simulink model "EPSAC_SM_BUCK"  (R2016a)
settings: Solver=VariableStepAuto  StartTime=0.0  StopTime=5  FixedStep=1e-5  RelTol=1e-3
libraries: powerlib x10
settings Model: Creator=jorda  LastModifiedBy=jorda

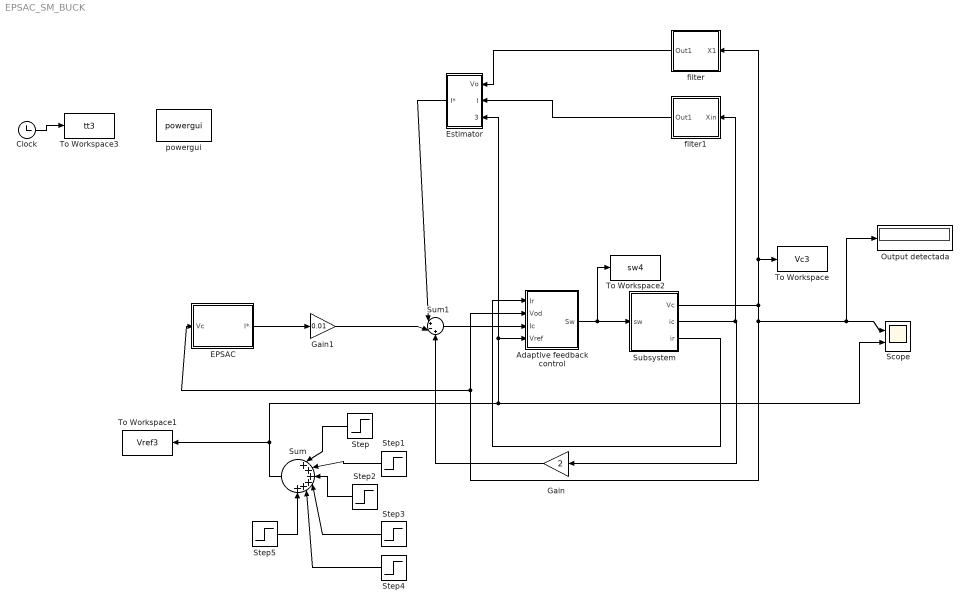
== system EPSAC_SM_BUCK ==
  "Adaptive feedback control " : Subsystem
  Clock : Clock
  EPSAC : Subsystem
  Estimator : Subsystem
  Gain : Gain  Gain=2
  Gain1 : Gain  Gain=0.01
  Output detectada : Display
  Scope : Scope  NumInputPorts=2
  Step : Step  Time=0.5  Before=3  After=4  SampleTime=0
  Step1 : Step  SampleTime=0
  Step2 : Step  Time=1.5  After=-2  SampleTime=0
  Step3 : Step  Time=2  After=-1  SampleTime=0
  Step4 : Step  Time=2.5  After=-1  SampleTime=0
  Step5 : Step  Time=3  After=2  SampleTime=0
  Subsystem : Subsystem
  Sum : Sum  Inputs=|++++++
  Sum1 : Sum  Inputs=|+-+
  To Workspace : ToWorkspace  VariableName=Vc3  SampleTime=1e-3
  To Workspace1 : ToWorkspace  VariableName=Vref3  SampleTime=1e-3
  To Workspace2 : ToWorkspace  VariableName=sw4  SampleTime=1e-3
  To Workspace3 : ToWorkspace  VariableName=tt3  SampleTime=1e-3
  filter : Subsystem
  filter1 : Subsystem
  powergui : powerlib/powergui  Priority=1  SimulationMode=Continuous  SolverType=Tustin/Backward Euler (TBE)  SampleTime=50e-6  frequency=60  SPID=off  DisableSnubberDevices=off  DisableRonSwitches=off  DisableVfSwitches=off  SwTol=0  DisplayEquations=off  Interpol=off  ExternalGateDelay=off  methode=off  Ts=10  FunctionMessages=off  echomessages=off  HookPort=off  EnableUseOfTLC=off  x0status=blocks  frequencyindice=0  Pbase=100e6  ErrMax=1e-4  Iterations=50  UnitsV=kV  UnitsW=MW  buscounter=0  RestoreLinks=warning  ResistiveCurrentMeasurement=off  Frange=[0:2:500]  Ylog=off  Xlog=on  ShowGrid=off  save=off  variable=ZData  structure=0  ZoomFFT=off  StartTime=0.0  cycles=1  DisplayStyle=1  fundamental=60  FreqAxis=off  MaxFrequency=1000  frequencyindicesteady=1  RmsSteady=1  display=off
  wires:
  "Adaptive feedback control "/1(Sw) -> To Workspace2/1, Subsystem/1("sw ")
  Step/1 -> Sum/1
  Step1/1 -> Sum/2
  Subsystem/3(ir) -> "Adaptive feedback control "/1(Ir)
  Sum1/1 -> "Adaptive feedback control "/3(Ic)
  Clock/1 -> To Workspace3/1
  EPSAC/1(I*) -> Gain1/1
  Step2/1 -> Sum/3
  Step3/1 -> Sum/4
  Step4/1 -> Sum/5
  Step5/1 -> Sum/6
  Gain/1 -> Sum1/3
  Gain1/1 -> Sum1/2
  Subsystem/1(Vc) -> Output detectada/1, Scope/1, "Adaptive feedback control "/2(Vod), EPSAC/1(Vc), filter/1(X1), To Workspace/1
  Sum/1 -> To Workspace1/1, Estimator/3(Vref), "Adaptive feedback control "/4(Vref), Scope/2
  Subsystem/2(ic) -> filter1/1(Xin), Gain/1
  filter/1(Out1) -> Estimator/1(Vo)
  filter1/1(Out1) -> Estimator/2(I)
  Estimator/1(I*) -> Sum1/1

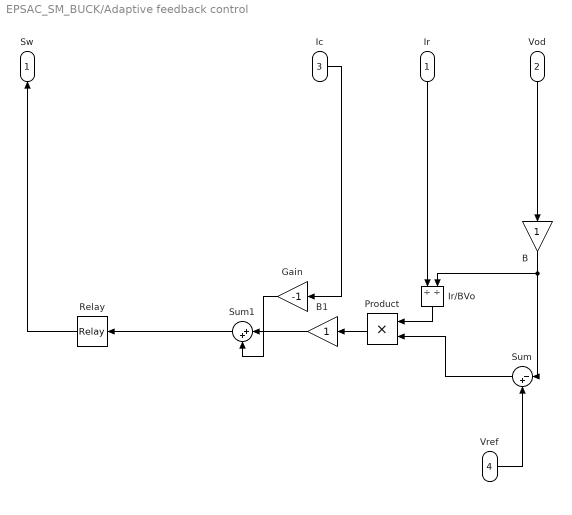
== system EPSAC_SM_BUCK/Adaptive feedback control  ==
  Ir : Inport
  Vod : Inport  Port=2
  Ic : Inport  Port=3
  Vref : Inport  Port=4
  B : Gain  ParamDataTypeStr=double  OutDataTypeStr=double
  B1 : Gain  ParamDataTypeStr=double  OutDataTypeStr=double
  Gain : Gain  Gain=-1  ParamDataTypeStr=double  OutDataTypeStr=double
  Ir/BVo : Product  Inputs=//
  Product : Product
  Relay : Relay  OnSwitchValue=0.6  OffSwitchValue=-0.6  OutDataTypeStr=double
  Sum : Sum  Inputs=|-+  AccumDataTypeStr=single  OutDataTypeStr=double  InputSameDT=on
  Sum1 : Sum  Inputs=|++  AccumDataTypeStr=double  OutDataTypeStr=double  InputSameDT=on
  Sw : Outport
  wires:
  Product/1 -> B1/1
  Ic/1 -> Gain/1
  Gain/1 -> Sum1/2
  Ir/1 -> Ir/BVo/1
  Ir/BVo/1 -> Product/1
  Vod/1 -> B/1
  B/1 -> Ir/BVo/2, Sum/1
  Sum/1 -> Product/2
  Vref/1 -> Sum/2
  Sum1/1 -> Relay/1
  Relay/1 -> Sw/1
  B1/1 -> Sum1/1

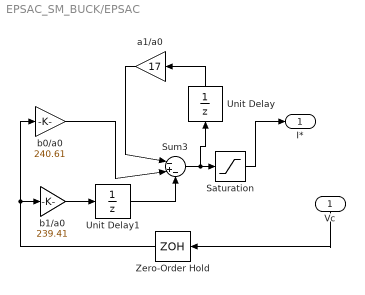
== system EPSAC_SM_BUCK/EPSAC ==
  Vc : Inport
  Saturation : Saturate  UpperLimit=1  LowerLimit=-1
  Sum3 : Sum  Inputs=|-+-
  Unit Delay : UnitDelay  SampleTime=1e-3
  Unit Delay1 : UnitDelay  SampleTime=1e-3
  Zero-Order Hold : ZeroOrderHold  SampleTime=1e-3
  a1/a0 : Gain  Gain=17
  b0/a0 : Gain  Gain=240.61
  b1/a0 : Gain  Gain=239.41
  I* : Outport
  wires:
  Vc/1 -> Zero-Order Hold/1
  Saturation/1 -> I*/1
  b0/a0/1 -> Sum3/2
  Zero-Order Hold/1 -> b0/a0/1, b1/a0/1
  b1/a0/1 -> Unit Delay1/1
  Unit Delay1/1 -> Sum3/3
  a1/a0/1 -> Sum3/1
  Unit Delay/1 -> a1/a0/1
  Sum3/1 -> Unit Delay/1, Saturation/1

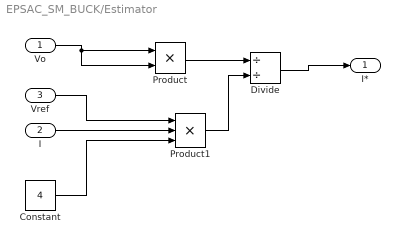
== system EPSAC_SM_BUCK/Estimator ==
  Vo : Inport
  I : Inport  Port=2
  Vref : Inport  Port=3
  Constant : Constant  Value=4
  Divide : Product  Inputs=//
  Product : Product
  Product1 : Product  Inputs=3
  I* : Outport
  wires:
  Divide/1 -> I*/1
  Product1/1 -> Divide/2
  Vo/1 -> Product/2, Product/1
  Product/1 -> Divide/1
  I/1 -> Product1/2
  Vref/1 -> Product1/1
  Constant/1 -> Product1/3

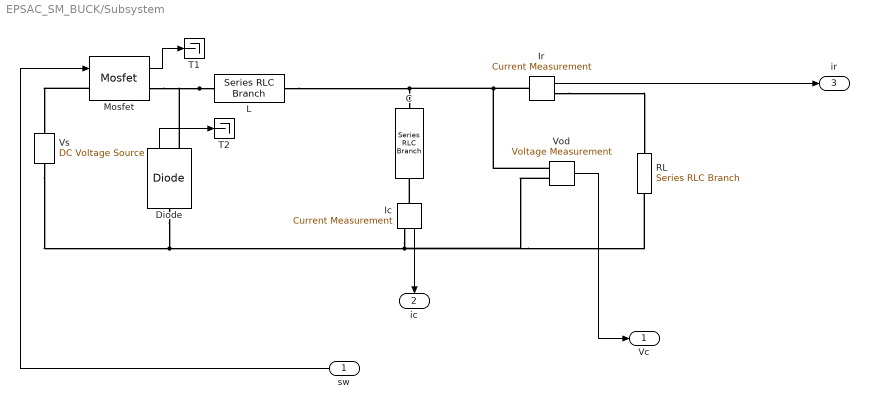
== system EPSAC_SM_BUCK/Subsystem ==
  "sw " : Inport
  C : powerlib/Elements/Series RLC Branch  LConnTagsString=__new0  RConnTagsString=__new0  BranchType=C  Resistance=1  Inductance=1e-3  SetiL0=off  InitialCurrent=0  Capacitance=2000e-6  Setx0=off  InitialVoltage=0  Measurements=None
  Diode : powerlib/Power Electronics/Diode  Ron=0.001  Lon=0  Vf=0.8  IC=0  UseSnubber=off  Rs=500  Cs=250e-9  Measurements=on
  Ic : powerlib/Measurements/Current Measurement  PhasorSimulation=off  OutputType=Complex  PSBequivalent=0
  Ir : powerlib/Measurements/Current Measurement  PhasorSimulation=off  OutputType=Complex  PSBequivalent=0
  L : powerlib/Elements/Series RLC Branch  LConnTagsString=__new0  RConnTagsString=__new0  BranchType=L  Resistance=1  Inductance=2e-3  SetiL0=off  InitialCurrent=0  Capacitance=1e-6  Setx0=off  InitialVoltage=0  Measurements=None
  Mosfet : powerlib/Power Electronics/Mosfet  Ron=0.1  Lon=0  Rd=0.01  Vfd=0  IC=0  Rs=1e5  Cs=inf  Measurements=on
  RL : powerlib/Elements/Series RLC Branch  LConnTagsString=__new0  RConnTagsString=__new0  BranchType=R  Resistance=4  Inductance=1e-3  SetiL0=off  InitialCurrent=0  Capacitance=1e-6  Setx0=off  InitialVoltage=0  Measurements=None
  T1 : Terminator
  T2 : Terminator
  Vod : powerlib/Measurements/Voltage Measurement  PhasorSimulation=off  OutputType=Complex  PSBequivalent=0
  Vs : powerlib/Electrical Sources/DC Voltage Source  Amplitude=15  Measurements=None
  Vc : Outport
  ic : Outport  Port=2
  ir : Outport  Port=3
  wires:
  "sw "/1 -> Mosfet/1
  Mosfet/1 -> T1/1
  Ic/1 -> ic/1
  Diode/1 -> T2/1
  Vod/1 -> Vc/1
  Ir/1 -> ir/1
  connections:
  Diode/LConn1 -- Vs/LConn1 -- Vod/LConn2 -- RL/RConn1 -- Ic/RConn1
  Ic/LConn1 -- C/RConn1
  Ir/LConn1 -- Vod/LConn1 -- L/RConn1 -- C/LConn1
  L/LConn1 -- Mosfet/RConn1 -- Diode/RConn1
  Ir/RConn1 -- RL/LConn1
  Mosfet/LConn1 -- Vs/RConn1

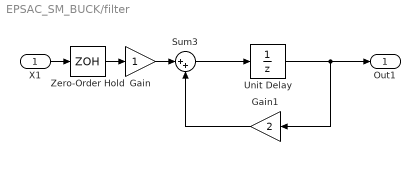
== system EPSAC_SM_BUCK/filter ==
  X1 : Inport
  Gain : Gain
  Gain1 : Gain  Gain=2
  Sum3 : Sum  Inputs=|++
  Unit Delay : UnitDelay  SampleTime=1e-3
  Zero-Order Hold : ZeroOrderHold  SampleTime=1e-3
  Out1 : Outport
  wires:
  Unit Delay/1 -> Out1/1, Gain1/1
  Zero-Order Hold/1 -> Gain/1
  Sum3/1 -> Unit Delay/1
  X1/1 -> Zero-Order Hold/1
  Gain/1 -> Sum3/1
  Gain1/1 -> Sum3/2

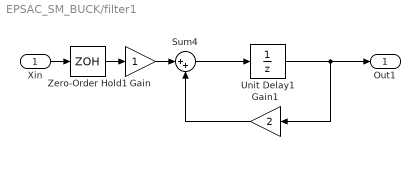
== system EPSAC_SM_BUCK/filter1 ==
  Xin : Inport
  Gain : Gain
  Gain1 : Gain  Gain=2
  Sum4 : Sum  Inputs=|++
  Unit Delay1 : UnitDelay  SampleTime=1e-3
  Zero-Order Hold1 : ZeroOrderHold  SampleTime=1e-3
  Out1 : Outport
  wires:
  Unit Delay1/1 -> Out1/1, Gain1/1
  Zero-Order Hold1/1 -> Gain/1
  Sum4/1 -> Unit Delay1/1
  Xin/1 -> Zero-Order Hold1/1
  Gain/1 -> Sum4/1
  Gain1/1 -> Sum4/2
